simulink model "PIC32MK_MCPWM_MCLV2_PIM_DualShunt_R2015b_InternalOpAmp"  (R2015b)
settings: Solver=FixedStepDiscrete  StartTime=0.0  StopTime=10.0  FixedStep=5e-5  RelTol=1e-3
undefined symbols (not defined in the file): A0, A11, A4, A8, AN0, AN24, AN3, AN9, B1, B6, B9, DiscIntNeverNeededParam, MaxPer, ms, Pin, PWM1max, Resol, us, XData
libraries: MCHP_Blockset x12, simulink x9
(part 1 of 2)
settings Model: Creator=M91449  LastModifiedBy=Lubin Kerhuel
settings DataIOCC: SaveFormat=Array  SignalLoggingSaveFormat=ModelDataLogs
settings OptimizationCC: DefaultParameterBehavior=Inlined  ExpressionDepthLimit=2147483647  OptimizeModelRefInitCode=on  LifeSpan=1
settings DebuggingCC: UnderspecifiedInitializationDetection=Classic  MergeDetectMultiDrivingBlocksExec=none  SolverPrmCheckMsg=warning  FcnCallInpInsideContextMsg=EnableAllAsWarning  StateNameClashWarn=warning
settings HardwareCC: ProdBitPerPointer=32  ProdLargestAtomicInteger=Integer  ProdWordSize=32  ProdLongLongMode=on  ProdHWDeviceType=Generic->Custom
settings ModelReferenceCC: ModelReferenceNumInstancesAllowed=Single
settings RTWCC: SystemTargetFile=MCHP_pic32_stf.tlc  TemplateMakefile=MCHP_pic32.tmf  Description=Microchip Embedded Target PIC32 (real-time)  GenerateReport=on  IncludeHyperlinkInReport=on  LaunchReport=on  GenerateTraceInfo=on  GenerateTraceReport=on  GenerateTraceReportSl=on  GenerateTraceReportSf=on  GenerateTraceReportEml=on  GenerateCodeReplacementReport=on
settings CodeAppCC: ForceParamTrailComments=on  IgnoreCustomStorageClasses=off  MaxIdLength=255  OperatorAnnotations=on  SimulinkDataObjDesc=on  SFDataObjDesc=on  MATLABFcnDesc=on  CustomSymbolStrType=$N$R$M  InsertBlockDesc=on  MATLABSourceComments=on  InternalIdentifier=Classic
settings STFCustomTargetCC: TargetLibSuffix=_lib.a  CodeReplacementLibrary=GNU C99 extensions  ConcurrentExecutionCompliant=off  IncludeMdlTerminateFcn=off  GeneratePreprocessorConditionals=Use local settings  CombineOutputUpdateFcns=on  CombineSignalStateStructs=on  SuppressErrorStatus=on  ERTCustomFileBanners=on  SupportAbsoluteTime=off  SupportNonFinite=off  SupportComplex=off  SupportContinuousTime=off  MATLABClassNameForMDSCustomization=Simulink.SoftwareTarget.ERTCustomization  CPPClassGenCompliant=off  GRTInterface=off  SystemTargetFile=MCHP_pic32_stf.tlc
settings ERTTargetCC: TargetLibSuffix=_lib.a  CodeReplacementLibrary=GNU C99 extensions  ParMdlRefBuildCompliant=off  CompOptLevelCompliant=off  ConcurrentExecutionCompliant=off  IncludeMdlTerminateFcn=off  CombineSignalStateStructs=on  SuppressErrorStatus=on  ERTFirstTimeCompliant=off  SupportAbsoluteTime=off  SupportNonFinite=off  SupportComplex=off  SupportNonInlinedSFcns=on  ModelStepFunctionPrototypeControlCompliant=off  CPPClassGenCompliant=off  UseToolchainInfoCompliant=off  InlinedParameterPlacement=NonHierarchical  ERTSrcFileBannerTemplate=MCHP_dsPIC_code_template.cgt  ERTHdrFileBannerTemplate=MCHP_dsPIC_code_template.cgt  ERTDataSrcFileTemplate=MCHP_dsPIC_code_template.cgt  ERTDataHdrFileTemplate=MCHP_dsPIC_code_template.cgt  ERTCustomFileTemplate=MCHP_main.tlc  ConvertIfToSwitch=on  SuppressUnreachableDefaultCases=on
settings ConfigComp: CovModelRefEnable=Off  CovSFcnEnable=off

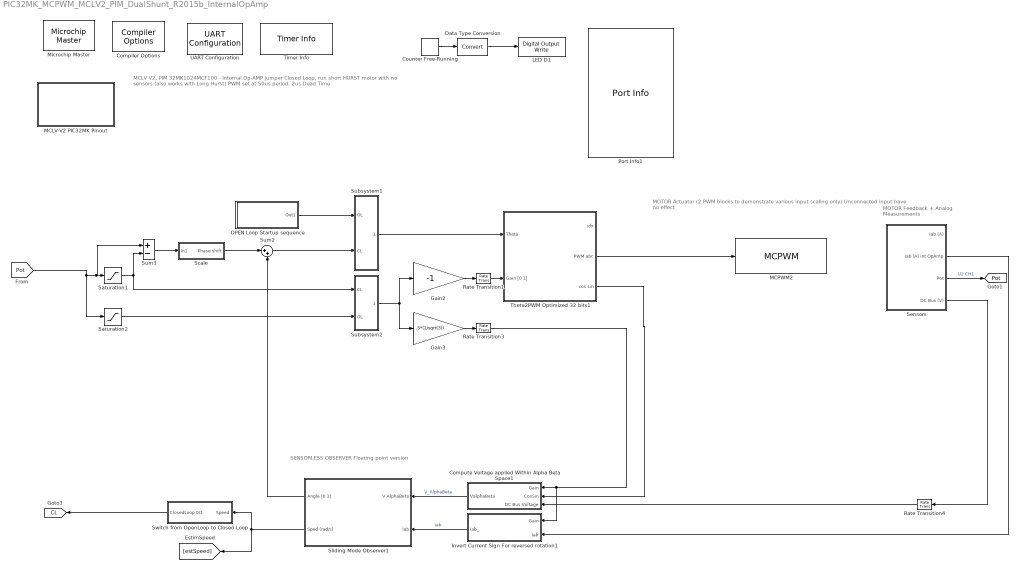
== system PIC32MK_MCPWM_MCLV2_PIM_DualShunt_R2015b_InternalOpAmp ==
  note: MOTOR Feedback
      | + Analog Measurements
  note: MOTOR Actuator (2 PWM blocks to demonstrate various input scaling only)
      | Unconnected input have no effect
  note: MCLV V2, PIM 32MK1024MCF100 - Internal Op-AMP jumper
      |
      | Closed Loop, run short HURST motor with no sensors (also works with Long Hurst)
      | PWM set at 50us period. 2us Dead Time
  note: SENSORLESS OBSERVER
      | Floating point version
  Compiler Options : MCHP_Blockset/System Configuration/Compiler Options  Priority=1  LATEST_CMPLR=on  COMP_LIST=Dynamic Options  COMP_LIST_TXT=xc32 - v2.41  DFP_LIST=Dynamic Options  DFP_LIST_TXT=v 1.4.94  CMSIS_DSP=Dynamic Options  CMSIS_DSP_TXT=Dynamic Options  USE_64BIT_DOUBLE=off  MCHP_MULTITHREAD_COMPILATION=on  UseCustom_LinkerScript=off  MCHP_MASTERLINK=PIC32MK_MCPWM_MCLV2_PIM_DualShunt_R2015b_InternalOpAmp/Microchip Master  OPTIMIZATION_LEVEL=1  OPTIMIZATION_FLTO=on  OPTIMIZATION_REORDER=off  UNROLL_LOOPS=on  PROCEDURAL_ABSTRACTION=off  MPLAB_LINKLIB=default  MPLAB_LINKLIB1=default  MCODE=is less than 32768 (faster)  MCONST=in code memory  MDATA=Use only memory below address 8192 (faster)  MSCALAR=Use only memory below address 8192 (faster)  MLARGEARRAY=off  MAGGREGATE=off  HEAP_SIZE=0  OMF=elf  DEBUG_INFO=on  ProduceHexOutput=on  AssemblyListing=on  NO_EDS_WARN=on  PRINT_STATISTICS=off
  Compute Voltage applied Within Alpha Beta Space1 : Subsystem
  Counter Free-Running : simulink/Sources/Counter Free-Running  NumBits=1  tsamp=.2
  Data Type Conversion : DataTypeConversion
  Gain2 : Gain  Gain=-1  OutMin=-PWM1max*0.5  OutMax=PWM1max*0.5  OutDataTypeStr=double  RndMeth=Zero
  Gain3 : Gain  Gain=.5*(2/sqrt(3))  OutDataTypeStr=double  RndMeth=Zero
  Invert Current Sign For reversed rotation1 : Subsystem
  LED D1 : MCHP_Blockset/Digital IO/Digital Output Write  PORT=Dynamic Options  PORT_TXT="F   [ 0  1  5  6  7  9  10  12  13 ]"  PIN=5  PACK=off  SIMULTANEOUS=off  ORDERING=None  SampleTime=-1  MCHP_PORT={Digital Out}{DOU}1:1:F5;  MCHP_MASTERLINK=PIC32MK_MCPWM_MCLV2_PIM_DualShunt_R2015b_InternalOpAmp/Microchip Master
  MCLV-V2 PIC32MK Pinout : Subsystem
  MCPWM2 : MCHP_Blockset/PWM IO/MCPWM  Priority=-2000  PWMx_ECAM_ITB=Independant - Center aligned - Symetric  PWMx_MTBS=Primary master timer  PWM_ClockResolution=Dynamic Options  PWM_ClockResolution_TXT=auto  MaxPeriod_s=50e-6  InitPeriode_s=50e-6  InitDutyCycleP_s=10e-6  InitDutyCycleS_s=10e-6  InitPhase_s=-1  SampleTime=-1  S_INPUT=[-1]  S_INPUT_Size=[3]  S_OUTPUT=[]  S_OUTPUT_Size=[]  S_ListCustomDatatype=S.S_ListCustomDatatype={};  MCHP_USER_INTERRUPTS=0  evalin_ws=PWM1max=MCHP_Fun.Hex2num('40A7700000000000');PWM2max=MCHP_Fun.Hex2num('40A7700000000000');PWM3max=MCHP_Fun.Hex2num('40A7700000000000');  MCHP_PORT={PWMH1 }{PWMH1}32:4:B14;{PWMH2 }{PWMH2}32:4:B12;{PWMH3 }{PWMH3}32:4:B10;{PWML1}{PWML1}32:4:B15;{PWML2}{PWML2}32:4:B13;{PWML3}{PWML3}32:4:B11;{PWM FLT15}{FLT15}32:0:B4;  MCHP_MASTERLINK=PIC32MK_MCPWM_MCLV2_PIM_DualShunt_R2015b_InternalOpAmp/Microchip Master  MCHP_CRC=3819763  PWMx_PMOD=Complementary  PWM1_HL=PWMxH & PWMxL output enabled  PWM1_swap=off  PWM1H_pol=off  PWM1L_pol=off  PWM2_HL=PWMxH & PWMxL output enabled  PWM2_swap=off  PWM2H_pol=off  PWM2L_pol=off  PWM3_HL=PWMxH & PWMxL output enabled  PWM3_swap=off  PWM3H_pol=off  PWM3L_pol=off  PWM4_HL=not used  PWM4_swap=off  PWM4H_pol=off  PWM4L_pol=off  PWM5_HL=not used  PWM5_swap=off  PWM5H_pol=off  PWM5L_pol=off  PWM6_HL=not used  PWM6_swap=off  PWM6H_pol=off  PWM6L_pol=off  PWM7_HL=not used  PWM7_swap=off  PWM7H_pol=off  PWM7L_pol=off  PWM8_HL=not used  PWM8_swap=off  PWM8H_pol=off  PWM8L_pol=off  PWM9_HL=not used  PWM9_swap=off  PWM9H_pol=off  PWM9L_pol=off  PWM10_HL=not used  PWM10_swap=off  PWM10H_pol=off  PWM10L_pol=off  PWM11_HL=not used  PWM11_swap=off  PWM11H_pol=off  PWM11L_pol=off  PWM12_HL=not used  PWM12_swap=off  PWM12H_pol=off  PWM12L_pol=off  Init_SEVTCMP_SSEVTCMP=-1  Init_TRIGx_STRIGx_1=[1.8e-6 ,-1]  Init_TRIGx_STRIGx_2=[-1 -1]  Init_TRIGx_STRIGx_3=[-1 -1]  Init_TRIGx_STRIGx_4=[-1 -1]  Init_TRIGx_STRIGx_5=[-1 -1]  Init_TRIGx_STRIGx_6=[-1 -1]  Init_TRIGx_STRIGx_7=[-1 -1]  Init_TRIGx_STRIGx_8=[-1 -1]  Init_TRIGx_STRIGx_9=[-1 -1]  Init_TRIGx_STRIGx_10=[-1 -1]  Init_TRIGx_STRIGx_11=[-1 -1]  Init_TRIGx_STRIGx_12=[-1 -1]  TRIG_DualTriggerMode=Primary Trigger to ADC is independant  BlockInput_VectorScalar=Vectors (grouped by function)  BlockInput_Period=Not a block input  BlockInput_DutyCycle=a Floating Point input within range [-1 1]  BlockInput_PhaseShift=Not a block input  BlockInput_SEVTCMP=Not a block input  BlockInput_TRIGx=Not a block input  BlockInput_DeadTime=Not a block input  BlockOutput_FaultDisabled=off  BlockOutput_Fault=off  DTC=Positive dead time (ensure period of time with PWM_H and PWM_L disasserted)  FLTSRC1_DTCMP=Dynamic Options  FLTSRC1_DTCMP_TXT="FLT6 / E13 / Pin[42]  -  Active HIGH"  FLTSRC2_DTCMP=Dynamic Options  FLTSRC2_DTCMP_TXT="FLT6 / E13 / Pin[42]  -  Active LOW"  FLTSRC3_DTCMP=Dynamic Options  FLTSRC3_DTCMP_TXT="FLT8 / E15 / Pin[44]  -  Active LOW"  FLTSRC4_DTCMP=Dynamic Options  FLTSRC4_DTCMP_TXT="FLT3 / C2 / Pin[34]  -  Active HIGH"  FLTSRC5_DTCMP=Dynamic Options  FLTSRC5_DTCMP_TXT="FLT3 / C2 / Pin[34]  -  Active HIGH"  FLTSRC6_DTCMP=Dynamic Options  FLTSRC6_DTCMP_TXT="FLT3 / C2 / Pin[34]  -  Active HIGH"  FLTSRC7_DTCMP=Dynamic Options  FLTSRC7_DTCMP_TXT="FLT3 / C2 / Pin[34]  -  Active HIGH"  FLTSRC8_DTCMP=Dynamic Options  FLTSRC8_DTCMP_TXT="FLT3 / C2 / Pin[34]  -  Active HIGH"  FLTSRC9_DTCMP=Dynamic Options  FLTSRC9_DTCMP_TXT="FLT3 / C2 / Pin[34]  -  Active HIGH"  FLTSRC10_DTCMP=Dynamic Options  FLTSRC10_DTCMP_TXT="FLT3 / C2 / Pin[34]  -  Active HIGH"  FLTSRC11_DTCMP=Dynamic Options  FLTSRC11_DTCMP_TXT="FLT3 / C2 / Pin[34]  -  Active HIGH"  FLTSRC12_DTCMP=Dynamic Options  FLTSRC12_DTCMP_TXT="FLT3 / C2 / Pin[34]  -  Active HIGH"  DeadTime_s=2e-6  DeadTimeAlt_s=2e-6  DeadTimeComp_s=0  FLTMODx=Force PWM output for current cycle. Enable PWM on next cycle  FLTSRCx=Dynamic Options  FLTSRCx_TXT="FLT15 / B4 / Pin[50]  -  Active LOW"  FLTDATx=PWM H/L -> 00  CLMODx=Disabled  CLSRCx=Dynamic Options  CLSRCx_TXT="FLT8 / E15 / Pin[44]  -  Active LOW"  CLDATx=PWM H/L -> 00  FLTLEBENx=off  CLLEBENx=off  LeadEdgeBlkPer_s=5e-7  PHRx=off  PHFx=off  PLRx=off  PLFx=off
  Microchip Master : MCHP_Blockset/System Configuration/Microchip Master  PICREF=32MK1024MCF100  TIMESTEP_REF=PWM1 trigger + ADC  BUSYFLAG=Dynamic Options  BUSYFLAG_TXT=None  PWRTEN=Not used  BOREN=Disable  BODENV=2.7V  BORV=Not used  FPWRT=128ms  DSBOREN=Enable ZPBOR during Deep Sleep Mode  DSLPBOR=Not used  MCLRE=Enabled  SMCLR=MCLR pin generates a normal system Reset  PMDL1WAY=Allow only one reconfiguration  RSTPRI=Device will obtain reset instruction from Primary flash  TEMP=Not used  SOSCSRC=Not used  SOSCSEL=Not used  IOL1WAY=Allow only one reconfiguration  ALTVREF=Not used  DISUVREG=Not used  DSSWEN=Not used  LPCFG=Not used  RTCBAT=Not used  VBTBOR=Not used  WUTSEL=Not used  POWERSAVE=off  FNOSC=Primary Osc (HS;EC)  FPR=ECIO w/ PLL 16x  FOSFPR=HS3 w/PLL 16x  FOS=Primary Oscillator  FRANGE=High Range  OSCILLATOR_SELECT=External Clock  OSCILLATOR_SELECT_spd=External Clock  QUARTZ=24e6  QUARTZ_spd=24e6  POSCGAIN=Gain Level 3 (highest)  POSCBOOST=Boost the kick start of the oscillator  SOSCGAIN=2x gain setting  SOSCBOOST=Boost the kick start of the oscillator  ACTIV_PLL=on  ACTIV_PLL_spd=on  MIPS_DESIRED=120e6  MIPS_DESIRED_spd=120e6  FPLLMUL=Not used  FPLLIDIV=1x Divider  POSCFREQ=Not used  POSCMD=EC (External Clock) Mode  POSCMOD=External clock mode  MIPS=120 * 1e6  ACLKCON=Optimized for PWM resolution & ADC conversion speed  ACLKCON_spd=Optimized for PWM resolution & ADC conversion speed  FPLLODIV=4x Divider  PLLKEN=Clock switch to PLL source will wait until the PLL lock signal is valid.  FCKSM=Clock Switch Enabled; FSCM Enabled  FCKSMEN=Sw Disabled; Mon Disabled  IESO=Enabled  DSWDTPS=1:2^36  FWDTEN=Disable  FWDTWINSZ=Window size is 25%  FWPSA=1:512  FWPSA0=1:128  FWPSB=1:16  WDT=Disable  WDTPOST=1:32768  WDTPRE=1:128  WDTPS=1:32768  WINDIS=Watchdog Timer is in non-Window mode  WWDTEN=Non-Window mode  DSWDTEN=Enable DSWDT during Deep Sleep Mode  DSWDTOSC=Select LPRC as DSWDT Reference clock  FPBDIV=Not used  FSOSCEN=Enable Secondary Oscillator  LPRCSEL=Not used  OSCIOFCN=Not used  OSCIOFNC=Disable  LVRCFG=Not used  PLL_96MHZ=Not used  PLL96MHZ=Not used  PLLDIV=Not used  WDTCLK=Not used  WDTCMX=Not used  WDTWIN=WDT Window is 25% of WDT period  XTCFG=24-32 MHz crystals  XTBST=Boost the kick-start  APL=Aux Flash Code protect is disabled  APLK=Aux Flash Write Protection or Code Protection is Enabled  AWRP=Auxiliary program memory is not write-protected  BSS=No Boot program Flash segment  BWP=Not used  BWRP=Boot Segment may be written  CP=Protection Disabled  EBS=No Boot EEPROM  ESS=No Segment Data EEPROM  GCP=General Segment Code protect is Disabled  GSS=General Segment Code protect is Disabled  GSS0=Not used  GSSK=General Segment Write Protection or Code Protection is Enabled  GWRP=General Segment may be written  PWP=Not used  RBS=No Boot RAM  RSS=No Secure RAM  SSS=No Secure Segment  SWRP=Secure segment may be written  WPCFG=Not used  WPDIS=Not used  WPEND=Not used  WPFP=Not used  ICESEL=Communicate on PGEC2/PGED2  ICS=Communicate on PGEC1 and PGED1  JTAGEN=Disable  COE=Not used  RES=Not used  DEBUG=Debugger is disabled  BACKBUG=Not used  BKBUG=Not used  ALTI2C=I2C mapped to SDA1/SCL1 pins  ALTI2C1=SDA1/SCK1 pins are selected as the I/O pins for I2C1  ALTI2C2=SDA2/SCK2 pins are selected as the I/O pins for I2C2  ALTI2C3=I2C3 mapped to SDA3/SCL3 pins  ALTQIO=QEA1; QEB1; INDX1 are selected as inputs to QEI1  ALTSS1=SS1A is selected as the I/O pin for SPI1  CMPPOL0=Hysteresis is applied to falling edge  CMPPOL1=Hysteresis is applied to falling edge  FCANIO=Not used  FETHIO=Default Ethernet I/O  FMIIEN=MII Enabled  FSRSSEL=Not used  FUSBIDIO=Controlled by the USB Module  FVBUSONIO=Not used  HPOL=PWM module high side output pins have active-high output polarity  HYST0=45 mV Hysteresis  HYST1=45 mV Hysteresis  I2C1SEL=Not used  LPOL=PWM module low side output pins have active-high output polarity  PWMPIN=PWM module pins controlled by PORT register at device Reset  RTCOSC=Not used  UPLLEN=USB PLL Enabled  UPLLIDIV=Not used  ATMOD8=Not used  ALTPMP=Not used  I2C2SEL=Not used  ALTADREF=Not used  ALTCVREF=Not used  PWMLOCK=PWM registers may be written without key sequence  INT_PRIORITY_DMA=0  MCHP_TIMER_RESULT=[ ]  MCHP_PLLRegisters="[34799619         0     16386         3        -1]"  MCHPVAR=MCHP.fcy.MIPS=1.2e+08;MCHP.fcy.SYSCLK=1.2e+08;MCHP.fcy.ADC=1.2e+08;MCHP.fcy.Comparator=1.2e+08;MCHP.fcy.I2C=1.2e+08;MCHP.fcy.SPI=1.2e+08;MCHP.fcy.UART=1.2e+08;MCHP.fcy.Timers=1.2e+08;MCHP.fcy.OC=1.2e+08;MCHP.fcy.IC=1.2e+08;MCHP.fcy.Ports=1.2e+08;MCHP.fcy.QEI=1.2e+08;MCHP.PowerSave=0;MCHP.TimeStepFactor=-20000;MCHP.TimeStep_Timer=-1;MCHP.NTIMERS=9;MCHP.id.name='32MK1024MCF100';MCHP.id.N=reshape([32 1024 100],1,3);MCHP.id.L=reshape({ 'MK','MCF',''},1,3);MCHP.id.Arch=4;MCHP.periph.PPS.reg_RPINRx=reshape(MCHP_Fun.Hex2num('[]'),0,0);MCHP.PPS.PIC32.PeriphInput_ppsGroup=reshape({ 'INT4','T2CK','T6CK','IC4','IC7','IC12','IC15','U3RX','U4CTS','U6RX','SDI1','SDI3','SCK4_in','SDI5','SS6_in','C3RX','REFCLKI','QEA1','HOME2','QEA3','HOME4','QEA5','HOME6','FLT1','23','24','25','26','27','28','29','30','31','INT3','T3CK','T7CK','IC3','IC8','IC11','IC16','U1CTS','U2RX','U5CTS','SDI2','SDI4','SCK4_in','C2RX','QEB1','INDX2','QEB3','INDX4','QEB5','INDX6','FLT2','SCK6_in','21','22','23','24','25','26','27','28','29','30','31','INT2','T4CK','T8CK','IC1','IC5','IC9','IC13','U1RX','U2CTS','U5RX','SS1_in','SS3_in','SS4_in','SS5_in','C1RX','OCFB','INDX1','QEB2','INDX3','QEB4','INDX5','QEB6','21','22','23','24','25','26','27','28','29','30','31','INT1','T5CK','T9CK','IC2','IC6','IC10','IC14','U3CTS','U4RX','U6CTS','SS2_in','SCK3_in','SCK5_in','SDI6','C4RX','OCFA','HOME1','QEA2','HOME3','QEA4','HOME5','QEA6','21','22','23','24','25','26','27','28','29','30','31'},1,132);MCHP.PPS.PIC32.PeriphOutputCode=reshape({ 'NoConnect','U1TX','U2RTS','SDO1','SDO2','OC1','OC7','C2OUT','C4OUT','OC13','10','U5RTS','C1TX','13','SDO3','SCK4_out','SDO5','SS6_out','REFOUT4','PTGTRIGO28','QEI1CNT','QEI5CNT','22','23','24','25','26','27','28','29','30','31','NoConnect','U3RTS','U4TX','SDO1','SDO2','OC2','OC8','C3OUT','OC9','OC12','OC16','U6RTS','C4TX','13','SDO2','SDO4','SDO5','SCK6_out','REFOUT3','PTGTRIGO29','QEI2CNT','QEI6CNT','22','23','24','25','26','27','28','29','30','31','NoConnect','U3TX','U4RTS','SS1_out','4','OC4','OC5','REFOUT1','C5OUT','OC10','OC14','U6TX','C3TX','13','SS3_out','SS4_out','SS5_out','SDO6','REFOUT2','19','QEI3CNT','21','22','23','24','25','26','27','28','29','30','31','NoConnect','U1RTS','U2TX','3','SS2_out','OC3','OC6','C1OUT','10','OC11','OC15','U5TX','C2TX','13','SCK3_out','SDO4','SCK5_out','SDO6','CTPLS','19','QEI4CNT','21','22','23','24','25','26','27','28','29','30','31'},1,128);MCHP.PPS.PIC32.PinInputCode=reshape({ 'A0','B3','B4','B15','B7','C7','C0','C5','A11','D5','G6','F1','E0','A15','CMP1','FHOME1','A1','B5','B1','B11','B8','A8','C8','B12','A12','D6','G7','G0','E1','A14','CMP2','FINDX1','B6','C15','A4','B13','B2','C6','C1','A7','E14','C13','G8','','F0','D4','PTGTRIGO30','FHOME2','B14','C12','B0','B10','B9','C9','C2','C4','E15','C10','G9','G12','G1','D3','PTGTRIGO31','FINDX2'},1,64);MCHP.Rx=reshape([22 24 32 -1 52 87 90 -1 -1 -1 -1 23 25 33 6 53 88 89 -1 -1 -1 -1 -1 26 34 7 -1 -1 -1 -1 -1 -1 -1 -1 27 -1 8 -1 -1 -1 -1 -1 -1 -1 51 50 -1 9 -1 -1 -1 -1 -1 -1 -1 -1 69 -1 82 -1 61 -1 -1 -1 -1 -1 -1 70 77 83 -1 91 10 -1 -1 -1 -1 3 72 78 -1 -1 92 11 -1 -1 -1 -1 49 74 81 68 18 -1 12 -1 -1 -1 -1 -1 76 84 -1 19 28 14 -1 -1 -1 -1 100 93 71 -1 -1 29 17 -1 -1 -1 -1 21 94 35 -1 -1 -1 38 -1 -1 -1 -1 20 98 63 79 41 40 96 -1 -1 -1 -1 -1 99 73 80 42 39 97 -1 -1 -1 -1 66 4 -1 47 43 -1 95 -1 -1 -1 -1 67 5 64 48 44 -1 1 -1 -1 -1 -1],11,16);MCHP.ADC.ANtype=reshape([0 0],1,2);MCHP.ADC.ADCONx=reshape([0 0 0 0 0 0],1,6);MCHP.ADC.ADCHS_0=reshape([0 0],1,2);MCHP.ADC.Flags=reshape([-1 0],1,2);MCHP.ADC.Buffer=reshape([-1 -1],1,2);MCHP.ADC.port=reshape([0 1 16 17 18 19 32 33 34 11 12 43 76 77 78 79 105 104 103 102 73 72 106 111 4 23 8 25 -1 -1 -1 -1 -1 89 90 107 93 92 62 63 64 65 -1 -1 -1 85 14 15 42 44 -1 -1 -1 -1 -1 -1 -1],1,57);MCHP.ADC.port_ALT=reshape([-1 -1 -1 -1],1,4);MCHP.ADC.port_VrefP=90;MCHP.ADC.port_VrefM=89;MCHP.ADC.port_AVdd=-1;MCHP.ADC.port_AVss=-1;MCHP.ADC.ADCDATA=reshape([1 1 1 1 1 1 1 1 1 1 1 1 1 1 1 1 1 1 1 1 1 1 1 1 1 1 1 1 0 0 0 0 0 1 1 1 1 1 1 1 1 1 0 0 0 1 1 1 1 1 1 1 1 1 0 0 0],1,57);MCHP.ADC.HS_SAR.TRGSRC=reshape([0 0 0 0 0 0 0 0 0 0 0 0 0 0 0 0 0 0 0 0 0 0 0 0 0 0],1,26);MCHP.ADC.HS_SAR.nFilters=0;MCHP.ADC.HS_SAR.nDedicatedCore=0;MCHP.ADC.HS_SAR.CALIBRATION=0;MCHP.ADC.HS_SAR.ADCON1L=-1;MCHP.ADC.HS_SAR.ADC_Class3_idxStart=32;MCHP.memory.RAM=0;MCHP.memory.RAM_XBegin=-1;MCHP.memory.RAM_YBegin=-1;MCHP.memory.RAM_dma=reshape([-1 -1],1,2);MCHP.memory.FLASH_ECC=0;MCHP.DMA.Num=8;MCHP.DMA.CNTmax=65535;MCHP.QEI.QEICONx=reshape([49023 49023 49023 49023 49023 49023],1,6);MCHP.QEI.QEItype=6;MCHP.QEI.Port_QEI_INDX=reshape([-1 -1],1,2);MCHP.QEI.Port_QEI_QEA=reshape([-1 -1],1,2);MCHP.QEI.Port_QEI_QEB=reshape([-1 -1],1,2);MCHP.QEI.Port_QEI_UPDN=reshape([-1 -1],1,2);MCHP.INT.Port=reshape([23 32767 32767 32767 32767],1,5);MCHP.PWM_HS.Flags=reshape([0 0 0],1,3);MCHP.PWM.port_FLT=reshape([-1 -1 -1 34 43 76 77 78 79 -1 -1 -1 -1 -1 -1 20 -1 -1 -1 -1 -1 -1 -1 -1 -1 -1 -1 -1 -1 -1 -1 -1 -1],1,33);MCHP.PWM.PWMRef=-1;MCHP.PWM.Flag=0;MCHP.PWM.Port_PWM_l=reshape([31 -1 29 -1 27 -1 7 -1 49 -1 51 -1 -1 -1 -1 -1 -1 -1 -1 -1 81 -1 54 -1],2,12);MCHP.PWM.Port_PWM_h=reshape([30 -1 28 -1 26 -1 10 -1 50 -1 52 -1 31 -1 29 -1 27 -1 7 -1 80 -1 53 -1],2,12);MCHP.PWM_HS_FEP.nEVTOUT=-1;MCHP.IC.Port=reshape([32767 32767 32767 32767 32767 32767 32767 32767 32767 32767 32767 32767 32767 32767 32767 32767],1,16);MCHP.IC.type=2;MCHP.OC.Port=reshape([32767 32767 32767 32767 32767 32767 32767 32767 32767 32767 32767 32767 32767 32767 32767 32767],1,16);MCHP.OC.type=2;MCHP.CN.Port=reshape([-1 -1 -1 -1 -1 -1 -1 -1 -1 -1 -1 -1 -1 -1 -1 -1 -1 -1 -1 -1 -1 -1 -1 -1 -1 -1 -1 -1 -1 -1 -1 -1 -1 -1 -1 -1 -1 -1 -1 -1 -1 -1 -1 -1 -1 -1 -1 -1 -1 -1 -1 -1 -1 -1 -1 -1 -1 -1 -1 -1 -1 -1 -1 -1 -1 -1 -1 -1 -1 -1 -1 -1 -1 -1 -1 -1 -1 -1 -1 -1 -1 -1 -1 -1 -1],1,85);MCHP.CN.PullUp=reshape([56723 65535 65479 61822 62211 14051 65475 0 0 0 0],1,11);MCHP.CN.type=2;MCHP.CN.Flag_PullDown=1;MCHP.SPI.Refs=reshape([1 2 3 4 5 6],1,6);MCHP.SPI.SPIxCON1=MCHP_Fun.Hex2num('41EFF07FFFE00000');MCHP.SPI.SPIxCON2=40843;MCHP.SPI.Port_SDI=reshape([-1 -1 -1 -1 -1 -1],1,6);MCHP.SPI.Port_SDO=reshape([-1 -1 -1 -1 -1 -1],1,6);MCHP.SPI.Port_SCK=reshape([23 22 -1 -1 -1 -1],1,6);MCHP.SPI.Port_SS=reshape([-1 -1 -1 -1 -1 -1],1,6);MCHP.I2C.Refs=reshape([1 2 3 4 0],1,5);MCHP.I2C.I2CxCON=8388607;MCHP.I2C.NewRegName=1;MCHP.I2C.Port_SDA=reshape([-1 -1 -1 -1 -1],1,5);MCHP.I2C.Port_SCL=reshape([-1 -1 -1 -1 -1],1,5);MCHP.I2C.Port_ASDA=reshape([-1 -1 -1 -1 -1],1,5);MCHP.I2C.Port_ASCL=reshape([-1 -1 -1 -1 -1],1,5);MCHP.I2C.Fuse_Port_SCL_SDA=reshape([-1 -1 -1 -1 -1 -1 -1 -1 -1 -1],2,5);MCHP.I2C.Fuse_Port_ASCL_ASDA=reshape([-1 -1 -1 -1 -1 -1 -1 -1 -1 -1],2,5);MCHP.SCCP.nSCCP=0;MCHP.SCCP.MCCP=reshape([0 0 0 0 0 0 0 0 0],1,9);MCHP.PGA.Port_PGA1P=reshape([-1 -1 -1 -1],1,4);MCHP.PGA.Port_PGA1N=reshape([-1 -1 -1 -1],1,4);MCHP.PGA.Port_PGA2P=reshape([-1 -1 -1 -1],1,4);MCHP.PGA.Port_PGA2N=reshape([-1 -1 -1 -1],1,4);MCHP.PGA.Num=0;MCHP.HS_AnalogComparator.Port_CMP1=reshape([-1 -1 -1 -1],1,4);MCHP.HS_AnalogComparator.Port_CMP2=reshape([-1 -1 -1 -1],1,4);MCHP.HS_AnalogComparator.Port_CMP3=reshape([-1 -1 -1 -1],1,4);MCHP.HS_AnalogComparator.Port_CMP4=reshape([-1 -1 -1 -1],1,4);MCHP.HS_AnalogComparator.PORT_EXTREFx=reshape([-1 -1],1,2);MCHP.HS_AnalogComparator.Port_DACOUTx=reshape([-1 -1],1,2);MCHP.HS_AnalogComparator.Num=0;MCHP.Comp.Port_CVrefin=-1;MCHP.Comp.Port_CVref=-1;MCHP.Comp.Port_CVref1O=-1;MCHP.Comp.Port_CVref2O=-1;MCHP.Comp.Port_CxOUT=reshape([32767 32767 32767 32767 32767],1,5);MCHP.Comp.Port_OAxOUT=reshape([17 0 32 -1 23],1,5);MCHP.Comp.Port_CxINP=reshape([18 1 34 32 4],1,5);MCHP.Comp.Port_CxINM=reshape([19 43 18 17 16 76 18 0 33 77 34 32 33 17 0 32 25 76 4 23],4,5);MCHP.Comp.Port_OAxINP=reshape([18 1 34 -1 4],1,5);MCHP.Comp.Port_OAxINM=reshape([19 16 33 -1 25],1,5);MCHP.Comp.nComp=reshape([5 0 0],1,3);MCHP.Comp.OpAmp=23;MCHP.Comp.CVRCON=reshape([0 0],1,2);MCHP.Comp.CMCON=0;MCHP.CDAC.Port_DACx=reshape([4 42 8],1,3);MCHP.CDAC.nCDAC=3;MCHP.UART.port_Rx=reshape([32767 32767 32767 32767 32767 32767],1,6);MCHP.UART.port_Tx=reshape([32767 32767 32767 32767 32767 32767],1,6);MCHP.UART.port_ARx=reshape([-1 -1],1,2);MCHP.UART.port_ATx=reshape([-1 -1],1,2);MCHP.UART.port_RTS=reshape([32767 32767 32767 32767 32767 32767],1,6);MCHP.UART.port_CTS=reshape([32767 32767 32767 32767 32767 32767],1,6);MCHP.UART.reg_UxMODE=reshape([13106175 13106175 13106175 13106175 13106175 13106175],1,6);MCHP.UART.reg_UxSTA=reshape(MCHP_Fun.Hex2num('[41EFFFFFFFE00000 41EFFFFFFFE00000 41EFFFFFFFE00000 41EFFFFFFFE00000 41EFFFFFFFE00000 41EFFFFFFFE00000]'),1,6);MCHP.modsrc.DOS_02551_cpu_16bit_v7=0;MCHP.modsrc.DOS_01520_wdt_dmt_upb_v1_16bit=0;MCHP.modsrc.DOS_02359a_sent_j2716_upb_v1=0;MCHP.modsrc.DOS_02672_math_progcrc_upb_v1_16bit=0;MCHP.modsrc.DOS_01577_cla_clc_upb_v1=0;MCHP.modsrc.DOS_02915_ecc_v2=0;MCHP.modsrc.DOS_02673_tmr_classa_upb_v1_16bit=0;MCHP.modsrc.DOS_01494_qei_32b_upb_v1_16bit=0;MCHP.modsrc.DOS_02552_msi_upb_v1_Master=0;MCHP.modsrc.DOS_01441_i2c_upb_v1_16bit_TLAH=0;MCHP.modsrc.DOS_03076_uart_protocol_upb_v1_16bit=0;MCHP.modsrc.DOS_01482=0;MCHP.modsrc.DOS_01483_pwm_16bit=0;MCHP.modsrc.DOS_02497_WACV=0;MCHP.modsrc.DOS_02316_nvm_ctrl_v1_16bit=0;MCHP.modsrc.DOS_02653_afe_current_bias_ctrl_upb_v1_16bit=0;MCHP.modsrc.DOS_01459_ptg_pc_upb_v1_16bit=0;MCHP.modsrc.DOS_01512_ccp_mccp_upb_v1_16bit=0;MCHP.modsrc.DOS_02519_dma_sfr_16bit_v2=0;MCHP.modsrc.DOS_02508c11=0;MCHP.modsrc.DOS_02475_dac_pdm_nbit_upb_v1_16bit=0;MCHP.modsrc.DOS_02467_gpio_upb_v1_16bit=0;MCHP.modsrc.DOS_00805_rst_integration_v4=0;MCHP.modsrc.DOS_02659_clk_sib_v12=0;MCHP.modsrc.DOS_02674_wdt_upb_v1_16bit=0;MCHP.modsrc.DOS_01407=0;MCHP.modsrc.DOS_02552_msi_upb_v1_Slave=0;MCHP.modsrc.DOS_02593_amp_pga_ctrl_pb_v2_16bit=0;MCHP.modsrc.DOS_03247_CAN_FD_UPB_V2_16_bit=0;MCHP.modsrc.DOS_01461_afe_ctmu_con_upb_v1_16bit=0;MCHP.modsrc.DOS_02497_WACA=0;MCHP.modsrc.DOS_02478_uart_irda_upb_v1_16bit=0;MCHP.modsrc.DOS_00929=0;MCHP.modsrc.DOS_01198=0;MCHP.modsrc.DOS_03029_WACH=0;MCHP.modsrc.DOS_02949_WACG=0;MCHP.modsrc.DOS_03349_amp_pad_opamp_ctrl_upb_v1=0;MCHP.modsrc.DOS_02237_osc_dco_ctrl_upb_v1_16bit=0;MCHP.modsrc.DOS_02472_ppi_pmp16_upb_v1_16bit=0;MCHP.modsrc.DOS_03994_WAC07=0;MCHP.modsrc.DOS_03662_WACU=0;MCHP.modsrc.DOS_00794=0;MCHP.modsrc.DOS_00931=0;MCHP.modsrc.DOS_00932=0;MCHP.modsrc.DOS_00942=0;MCHP.modsrc.DOS_00938=0;MCHP.modsrc.DOS_00996=0;MCHP.modsrc.DOS_00997=0;MCHP.modsrc.DOS_00998=0;MCHP.modsrc.DOS_00209=0;MCHP.modsrc.DOS_01555_adc=0;MCHP.modsrc.DOS_01293=0;MCHP.modsrc.DOS_00828=0;MCHP.modsrc.DOS_01116=0;MCHP.modsrc.DOS_01017_RPORx=0;MCHP.modsrc.DOS_01017_RPINRx=0;MCHP.modsrc.DOS_01555_nvm_tsmc18_v2_16bit=0;MCHP.modsrc.DOS_00804=0;MCHP.modsrc.DOS_00826=0;MCHP.modsrc.DOS_01555_TLAK_PMDx=0;MCHP.modsrc.DOS_01555_TLAK_INT_=0;MCHP.modsrc.DOS_00933=0;MCHP.modsrc.DOS_01555=0;MCHP.modsrc.DOS_01555_ptg=0;MCHP.modsrc.DOS_00958=0;MCHP.modsrc.DOS_01117_PORTx=0;MCHP.modsrc.DOS_00999=0;MCHP.modsrc.DOS_01041=0;MCHP.modsrc.DOS_00892=0;MCHP.modsrc.DOS_01287_TLAC_PMDx=0;MCHP.modsrc.DOS_01287_TLAC_INT_=0;MCHP.modsrc.DOS_01424=0;MCHP.modsrc.DOS_01332=0;MCHP.modsrc.DOS_01468_PMBA_current_source=0;MCHP.modsrc.DOS_02291_PGA=0;MCHP.modsrc.DOS_01467_Comparator=0;MCHP.modsrc.DOS_01498_TLAY=0;MCHP.modsrc.DOS_00993_PLL_120MHz=0;MCHP.modsrc.DOS_01332_ptg_pc_v1=0;MCHP.modsrc.DOS_00958_pwm_TLAY=0;MCHP.modsrc.TLAY_IOPorts=0;MCHP.modsrc.DOS_00929q=0;MCHP.modsrc.DOS_02415_spi_v5=0;MCHP.modsrc.DOS_RPINRx_16bit_2=0;MCHP.modsrc.DOS_01497_TLAH_PMDx=0;MCHP.modsrc.DOS_02550_TLAL_INT=0;MCHP.modsrc.DOS_00958_pwm_TLAH=0;MCHP.modsrc.DOS_01287_TLAH_INT_=0;MCHP.modsrc.DOS_01113=0;MCHP.modsrc.DOS_01017_PMDx=0;MCHP.modsrc.DOS_00927=0;MCHP.modsrc.DOS_01080=0;MCHP.modsrc.DOS_00794_cpu_16bit_v3=0;MCHP.modsrc.DOS_02192_TLCD_PMDx=0;MCHP.modsrc.DOS_02192_TLCD_INT_=0;MCHP.modsrc.DOS_02192_cmp=0;MCHP.modsrc.DOS_00958_pwm_TLCD=0;MCHP.modsrc.DOS_02192_PORTx_TLCD=0;MCHP.modsrc.DOS_00936=0;MCHP.modsrc.DOS_00995=0;MCHP.modsrc.DOS_00546=0;MCHP.modsrc.DOS_00474=0;MCHP.modsrc.DOS_02481_WACJ_MC_Config=1;MCHP.modsrc.DOS_02569_pfm_cache_ocp_v1=1;MCHP.modsrc.DOS_02819_pfm_ctrl_32bit_upb_v2=1;MCHP.modsrc.DOS_02674_wdt_upb_v1_32bit=1;MCHP.modsrc.DOS_01520_wdt_dmt_upb_v1=1;MCHP.modsrc.DOS_02869_icd_jtag_bvci_upb_v2=1;MCHP.modsrc.DOS_02823_WACJ_clk_cru_upb_v2=1;MCHP.modsrc.DOS_01423_RPINRx=1;MCHP.modsrc.DOS_02481_RPORx=1;MCHP.modsrc.DOS_02511_pwr_sib_upb_v1_32bit=1;MCHP.modsrc.DOS_02481_WACJ_MC_int_evic_v3=1;MCHP.modsrc.DOS_01500_dma_bvci_v2=1;MCHP.modsrc.DOS_02141_tmr_classa_pb_v2=1;MCHP.modsrc.DOS_02815_tmr_classb_upb_v1=1;MCHP.modsrc.DOS_00740_icap_pb_v1=1;MCHP.modsrc.DOS_00749_ocmp_pb_v1=1;MCHP.modsrc.DOS_01441_i2c_upb_v1_32bit=1;MCHP.modsrc.DOS_01329_spi_pb_v2=1;MCHP.modsrc.DOS_02478_uart_irda_upb_v1_32bit=1;MCHP.modsrc.DOS_02514_dfm_strl_sst_upb_v1=1;MCHP.modsrc.DOS_01477_pwm_mc_upb_v1=1;MCHP.modsrc.DOS_01459_ptg_pc_upb_v1_SIC=1;MCHP.modsrc.DOS_01494_qei_32b_upb_v1=1;MCHP.modsrc.DOS_01427_cmp_control_upb_v1_32bit=1;MCHP.modsrc.DOS_01445_dac_nbit__control_upb_v1_32bit=1;MCHP.modsrc.DOS_01461_afe_ctmu_con_upb_v1=1;MCHP.modsrc.DOS_02472_ppi_pmp16_upb_v1=1;MCHP.modsrc.DOS_02467_gpio_ports_upb_v1=1;MCHP.modsrc.DOS_01152_can_bvci_v1=1;MCHP.modsrc.DOS_02508_adc_sar_ctrl_upb_v1_PIC32MK=1;MCHP.modsrc.DOS_02813a_usb_otgcore_pb_v3=1;MCHP.modsrc.DOS_01261_tmr_rtcc_pb_v2=1;MCHP.modsrc.DOS_01475_lpwr_deep_sleep_ctrl_v2=1;MCHP.modsrc.DOS_EIP_00136_ssx_v1=1;MCHP.modsrc.DOS_02481_WACK_MC_Config=0;MCHP.modsrc.DOS_03088_pfm_cache_ocp_v2_WACK=0;MCHP.modsrc.DOS_02823_WACN_clk_cru_upb_v2=0;MCHP.modsrc.DOS_02907_WACK_MC_int_evic_v3=0;MCHP.modsrc.DOS_03554_cmp_control_upb_v2_32bit=0;MCHP.modsrc.DOS_03247_can_fd_upb_v2_pic32mk=0;MCHP.modsrc.DOS_02787_WACD_Config=0;MCHP.modsrc.DOS_00800_dac_4bit_ctrl_pb_v1=0;MCHP.modsrc.DOS_01539_icd_jtag_pb_v2=0;MCHP.modsrc.DOS_02823_clk_cru_upb_v2=0;MCHP.modsrc.DOS_01423_RPORx=0;MCHP.modsrc.DOS_02907_WACD_int_evic_v3=0;MCHP.modsrc.DOS_00734_uart_irda_pb_v1=0;MCHP.modsrc.DOS_00687_tmr_classa_pb_v1=0;MCHP.modsrc.DOS_00745_tmr_classb_pb_v1=0;MCHP.modsrc.DOS_02508_adc_sar_ctrl_upb_v1=0;MCHP.modsrc.DOS_00866_cmp_control_pb_v2=0;MCHP.modsrc.DOS_01114_eth_bvci_v1=0;MCHP.modsrc.DOS_02831_usb_clk_rst_v2=0;MCHP.modsrc.DOS_01643_pfm_cache_ahb_v2=0;MCHP.modsrc.DOS_EIP_00206r5_sqi_v2=0;MCHP.modsrc.DOS_EIP_00124_usb_hs_otgcore_v1=0;MCHP.modsrc.DOS_EIP_00218_math_rng_ahbs_v2=0;MCHP.modsrc.DOS_EIP_00109_ebi_v1=0;MCHP.modsrc.DOS_EIP_00158_crypto_v1=0;MCHP.PortBase=16;MCHP.PortPrefixe='P';MCHP.clock.PBxDIV=reshape([0 0 0 0 0 3 0 -1],1,8);  MCHP_CRC=15127327  BTMODE=Not used  RES1=Not used  PLLSS=Not used  RES2=Not used  ALTCMPI=Not used  BOREN1=Not used  ALTRB6=Not used  RETCFG=Not used  DFMCY=Not used  BSS2=No Boot Segment  BSEN=No Boot Segment  CWRP=Configuration Segment may be written  CSS=No Protection (other than CWRP)  AIVTDIS=Disable Alternate Vector Table  BSLIM=Not used  WDTEN=Disable  BTSWP=BOOTSWP instruction is disabled  DBCC=No Cross Connection between DAC outputs  CTXT1=Not Assigned  CTXT2=Not Assigned  SEQNUM=Not used  nSEQNUM=Not used  BOREN0=Enabled  DMTIVT=Not used  DMTCNT=2^31 (2147483648)  DMTEN=Dead Man Timer is Enabled and cannot be disabled by software  ON=Not used  USERID=Not used  RESERVED1=Not used  PGL1WAY=Allow only one reconfiguration  FPLLRNG=13-26 MHz Input  FPLLICLK=POSC is input to the System PLL  FPLLMULT=PLL Multiply by 20  UPLLFSEL=USB PLL input is 24 MHz  DMTINTV=Window/Interval value is 127/128 counter value  WDTSPGM=WDT stops during Flash programming  FDMTEN=Deadman Timer is disabled  TRCEN=Trace features in the CPU are enabled  BOOTISA=Boot code and Exception code is MIPS32  FECCCON=ECC and Dynamic ECC are disabled (ECCCON bits are writable)  EXTDDRSIZE=Not used  FSLEEP=Flash is powered down when the device is in Sleep mode  DBGPER=Allow CPU access to all permission regions  EJTAGBEN=Normal EJTAG functionality  TSEQ=Not used  CSEQ=Not used  RWDTPS=1:1048576  RCLKSEL=Always use LPRC  SWDTPS=1:1048576  DMTIVTL=Not used  DMTIVTH=Not used  DMTCNTL=Not used  DMTCNTH=Not used  DMTDIS=Dead Man Timer is Disabled and can be enabled by software  SMBEN=SMBus input threshold is enabled  SPI2PIN=SPI2 uses I/O remap (PPS) pins  CTXT3=Not Assigned  CTXT4=Not Assigned  MBXM0=Mailbox register configured for Master data read (Slave to Master data transfer)  MBXM1=Mailbox register configured for Master data read (Slave to Master data transfer)  MBXM2=Mailbox register configured for Master data read (Slave to Master data transfer)  MBXM3=Mailbox register configured for Master data read (Slave to Master data transfer)  MBXM4=Mailbox register configured for Master data read (Slave to Master data transfer)  MBXM5=Mailbox register configured for Master data read (Slave to Master data transfer)  MBXM6=Mailbox register configured for Master data read (Slave to Master data transfer)  MBXM7=Mailbox register configured for Master data read (Slave to Master data transfer)  MBXM8=Mailbox register configured for Master data read (Slave to Master data transfer)  MBXM9=Mailbox register configured for Master data read (Slave to Master data transfer)  MBXM10=Mailbox register configured for Master data read (Slave to Master data transfer)  MBXM11=Mailbox register configured for Master data read (Slave to Master data transfer)  MBXM12=Mailbox register configured for Master data read (Slave to Master data transfer)  MBXM13=Mailbox register configured for Master data read (Slave to Master data transfer)  MBXM14=Mailbox register configured for Master data read (Slave to Master data transfer)  MBXM15=Mailbox register configured for Master data read (Slave to Master data transfer)  MBXHSA=MSIxMBXD15 assigned to mailbox handshake protocol block A  MBXHSB=MSIxMBXD15 assigned to mailbox handshake protocol block B  MBXHSC=MSIxMBXD15 assigned to mailbox handshake protocol block C  MBXHSD=MSIxMBXD15 assigned to mailbox handshake protocol block D  MBXHSE=MSIxMBXD15 assigned to mailbox handshake protocol block E  MBXHSF=MSIxMBXD15 assigned to mailbox handshake protocol block F  MBXHSG=MSIxMBXD15 assigned to mailbox handshake protocol block G  MBXHSH=MSIxMBXD15 assigned to mailbox handshake protocol block H  HSAEN=Mailbox data flow control handshake protocol block disabled.  HSBEN=Mailbox data flow control handshake protocol block disabled.  HSCEN=Mailbox data flow control handshake protocol block disabled.  HSDEN=Mailbox data flow control handshake protocol block disabled.  HSEEN=Mailbox data flow control handshake protocol block disabled.  HSFEN=Mailbox data flow control handshake protocol block disabled.  HSGEN=Mailbox data flow control handshake protocol block disabled.  HSHEN=Mailbox data flow control handshake protocol block disabled.  CPRA0=Master core owns pin.  CPRA1=Master core owns pin.  CPRA2=Master core owns pin.  CPRA3=Master core owns pin.  CPRA4=Master core owns pin.  CPRB0=Master core owns pin.  CPRB1=Master core owns pin.  CPRB2=Master core owns pin.  CPRB3=Master core owns pin.  CPRB4=Master core owns pin.  CPRB5=Master core owns pin.  CPRB6=Master core owns pin.  CPRB7=Master core owns pin.  CPRB8=Master core owns pin.  CPRB9=Master core owns pin.  CPRB10=Master core owns pin.  CPRB11=Master core owns pin.  CPRB12=Master core owns pin.  CPRB13=Master core owns pin.  CPRB14=Master core owns pin.  CPRB15=Master core owns pin.  CPRC0=Master core owns pin.  CPRC1=Master core owns pin.  CPRC2=Master core owns pin.  CPRC3=Master core owns pin.  CPRC4=Master core owns pin.  CPRC5=Master core owns pin.  CPRC6=Master core owns pin.  CPRC7=Master core owns pin.  CPRC8=Master core owns pin.  CPRC9=Master core owns pin.  CPRC10=Master core owns pin.  CPRC11=Master core owns pin.  CPRC12=Master core owns pin.  CPRC13=Master core owns pin.  CPRC14=Master core owns pin.  CPRC15=Master core owns pin.  CPRD0=Master core owns pin.  CPRD1=Master core owns pin.  CPRD2=Master core owns pin.  CPRD3=Master core owns pin.  CPRD4=Master core owns pin.  CPRD5=Master core owns pin.  CPRD6=Master core owns pin.  CPRD7=Master core owns pin.  CPRD8=Master core owns pin.  CPRD9=Master core owns pin.  CPRD10=Master core owns pin.  CPRD11=Master core owns pin.  CPRD12=Master core owns pin.  CPRD13=Master core owns pin.  CPRD14=Master core owns pin.  CPRD15=Master core owns pin.  CPRE0=Master core owns pin.  CPRE1=Master core owns pin.  CPRE2=Master core owns pin.  CPRE3=Master core owns pin.  CPRE4=Master core owns pin.  CPRE5=Master core owns pin.  CPRE6=Master core owns pin.  CPRE7=Master core owns pin.  CPRE8=Master core owns pin.  CPRE9=Master core owns pin.  CPRE10=Master core owns pin.  CPRE11=Master core owns pin.  CPRE12=Master core owns pin.  CPRE13=Master core owns pin.  CPRE14=Master core owns pin.  CPRE15=Master core owns pin.  S1FNOSC=Internal Fast RC (FRC) Oscillator with postscaler  S1IESO=Start up with FRC; then switch  S1OSCIOFNC=OSC2 is clock output  S1FCKSM=Both Clock switching and Fail-safe Clock Monitor are disabled  S1PLLKEN=S1PLLKEN_ON  S1RWDTPS=1:1048576  S1RCLKSEL=Always use LPRC  S1WINDIS=Watchdog Timer operates in Non-Window mode  S1WDTWIN=WDT Window is 25% of WDT period  S1SWDTPS=1:1048576  S1FWDTEN=Disable  S1ICS=Communicate on PGC1 and PGD1  S1DEBUG=Not used  S1ISOLAT=The slave can operate (in debug mode) even if the SLVEN bit in the MSI is zero.  S1NOBTSWP=BOOTSWP instruction is disabled  S1ALTI2C1=I2C1 mapped to SDA1/SCL1 pins  S1SPI1PIN=Slave SPI1 uses I/O remap (PPS) pins  S1SSRE=Slave generated resets will reset the Slave Enable Bit in the MSI module  S1MSRE=The master software oriented RESET events (RESET Op-Code; Watchdog timeout; TRAP reset; illegalInstruction) will also cause the slave subsystem to reset.  S1CTXT1=Not Assigned  S1CTXT2=Not Assigned  S1CTXT3=Not Assigned  S1CTXT4=Not Assigned  BORLVL=Not used  BSSO=Not used  MCA=Not used  MAXTEMP=Not used  CFGAN14=Not used  CFGAN15=Not used  S1IOL1WAY=Not used  S1BSSO=Not used  S1BACKBUG=Not used  BISTDIS=mBIST on reset feature disabled  NOBTSWP=BOOTSWP instruction is disabled  S1BISTDIS=Slave BIST on reset feature disabled  S1DMTIVTL=Not used  S1DMTIVTH=Not used  S1DMTCNTL=Not used  S1DMTCNTH=Not used  S1DMTDIS=Slave Dead Man Timer is Disabled and can be enabled by software  BSEQ=Not used  IBSEQ=Not used  SMB3EN=SMBus 3.0 input levels  FUSBIDIO2=USBID pin is controlled by the USB2 module  FVBUSIO2=VBUSON pin is controlled by the USB2 module  FUSBIDIO1=USBID pin is controlled by the USB1 module  FVBUSIO1=VBUSON pin is controlled by the USB1 module  VBATBOREN=Enable ZPBOR during VBAT Mode  FDSEN=Enable DSEN bit in DSCON  BORSEL=BOR trip voltage 2.1v (Non-OPAMP deviced operation)  POSCFGAIN=Gain is G3  POSCAGCDLY=Settling time = 25ms x AGCRNG  POSCAGCRNG=Range 1x  POSCAGC=Automatic Gain Control for Oscillator  FDBGWP=Not used
  OPEN Loop Startup sequence : Subsystem
  Port Info1 : MCHP_Blockset/System Info/Port Info  MCHP_MASTERLINK=PIC32MK_MCPWM_MCLV2_PIM_DualShunt_R2015b_InternalOpAmp/Microchip Master
  Rate Transition1 : RateTransition
  Rate Transition3 : RateTransition
  Rate Transition4 : RateTransition  Deterministic=off
  Saturation1 : Saturate  UpperLimit=sqrt(3)/2 * (49/50)  LowerLimit=-sqrt(3)/2 * (49/50)
  Saturation2 : Saturate  UpperLimit=0.84*.3  LowerLimit=-0.84*.3
  Scale : Subsystem
  Sensors : Subsystem
  Sliding Mode Observer1 : Subsystem
  Subsystem1 : Subsystem
  Subsystem2 : Subsystem
  Sum2 : Sum  Inputs=|++
  Sum3 : Sum  Inputs=+-
  Switch from OpenLoop to Closed Loop : Subsystem
  Theta2PWM Optimized 32 bits1 : Subsystem  VariantControl=Optimized
  Timer Info : MCHP_Blockset/System Info/Timer Info  MCHP_MASTERLINK=PIC32MK_MCPWM_MCLV2_PIM_DualShunt_R2015b_InternalOpAmp/Microchip Master
  UART Configuration : MCHP_Blockset/BUS UART/UART Configuration  UART_REF=2  BAUD_Choice=Dynamic Options  BAUD_Choice_TXT="6000000         [+0.00%]"  BAUD_Choice_IR=Dynamic Options  BAUD_Choice_IR_TXT=[]  BAUD_Custom=115200  INT_PRIORITY=0  ALT_IO=on  PIN_RX=Dynamic Options  PIN_RX_TXT=A8 / Pin[49]  PIN_TX=Dynamic Options  PIN_TX_TXT=B9 / Pin[76]  MCHP_PORT="{UART2  Rx}{U2RX}3:0:P8;{UART2  Tx}{U2TX}3:1:P25;"  MCHP_MASTERLINK=PIC32MK_MCPWM_MCLV2_PIM_DualShunt_R2015b_InternalOpAmp/Microchip Master  MCHP_COM_ExtPil=off  TX_IMPLEMENTATION=Circular Buffer  TX_IMPLEMENTATION_default=Circular Buffer  TX_INT_PRIORITY=5  TX_INT_WHEN=is empty & last char is sent  TX_INT_WHEN_default=is empty & last char is sent  TX_CIRCULAR_SIZE=256  TX_DMA_CHANNEL="0   (Lowest Priority)"  TX_DMA_SIZE=[]  TX_TASK_PROTECTION=Delay tasks (default)  TX_INTERRUPT_PROTECTION=Do not send on conflict (default)  TX_INTERRUPT_PROTECTION_default=Do not send on conflict (default)  RX_IMPLEMENTATION=Circular Buffer  RX_IMPLEMENTATION_default=Circular Buffer  RX_INT_PRIORITY=1  RX_INT_WHEN=receive 1 character  RX_CIRCULAR_SIZE=256  RX_DMA_CHANNEL=0  RX_DMA_SIZE=0  DuplexMode=Full duplex (default)  PIN_RX_Inv=off  PIN_TX_Inv=off  PIN_RXTX_Inv=off  ParityBit=No parity (default)  StopBit=1 stop bit (default)  IRDA=off  FlowControl=None  PIN_CTS=Dynamic Options  PIN_CTS_TXT=B6 / Pin[70]  PIN_RTS=Dynamic Options  PIN_RTS_TXT=A0 / Pin[22]  InitSequence_chkbox=off  BAUD_Choice_InitSeq=Dynamic Options  BAUD_Choice_InitSeq_TXT="110         [+4.04%]"  BAUD_Choice_IR_InitSeq=Dynamic Options  BAUD_Choice_IR_InitSeq_TXT=0  BAUD_Custom_InitSeq=0  InitSequence='Hello World'
  tag scope: CL=global, Pot=global
  wires:
  Theta2PWM Optimized 32 bits1/2(PWM abc) -> MCPWM2/1
  Sliding Mode Observer1/2(Sped (rad/s)) -> Switch from OpenLoop to Closed Loop/1(Speed), [estSpeed]
  Sliding Mode Observer1/1(Angle [0 1]) -> Sum2/2
  Sensors/3(Pot) -> [Pot]  "U2 CH1"
  Subsystem1/1(OL/CL) -> Theta2PWM Optimized 32 bits1/1(Theta)
  Subsystem2/1(OL/CL) -> Gain2/1, Gain3/1
  Gain2/1 -> Rate Transition1/1
  Gain3/1 -> Rate Transition3/1
  Saturation1/1 -> Sum3/2, Subsystem2/1(CL)
  Saturation2/1 -> Subsystem2/2(OL)
  Rate Transition1/1 -> Theta2PWM Optimized 32 bits1/2(Gain [0 1])
  Switch from OpenLoop to Closed Loop/1(ClosedLoop 0/1) -> [CL]
  [Pot] -> Saturation2/1, Sum3/1, Saturation1/1
  Sum2/1 -> Subsystem1/2(CL)
  OPEN Loop Startup sequence/1(Out1) -> Subsystem1/1(OL)
  Sum3/1 -> Scale/1(In1)
  Scale/1(Phase shift) -> Sum2/1
  Counter Free-Running/1 -> Data Type Conversion/1
  Data Type Conversion/1 -> LED D1/1
  Invert Current Sign For reversed rotation1/1("Iab_ ") -> Sliding Mode Observer1/2(Iab)  "Iab"
  Compute Voltage applied Within Alpha Beta Space1/1(ValphaBeta) -> Sliding Mode Observer1/1(V AlphaBeta)  "V_AlphaBeta"
  Rate Transition3/1 -> Invert Current Sign For reversed rotation1/1(Gain), Compute Voltage applied Within Alpha Beta Space1/1(Gain)
  Theta2PWM Optimized 32 bits1/3(cos sin) -> Compute Voltage applied Within Alpha Beta Space1/2(CosSin)
  Rate Transition4/1 -> Compute Voltage applied Within Alpha Beta Space1/3(DC Bus Voltage)
  Sensors/2(Iab (A) int OpAmp) -> Invert Current Sign For reversed rotation1/2("Iab ")
  Sensors/4(DC Bus (V)) -> Rate Transition4/1

== system PIC32MK_MCPWM_MCLV2_PIM_DualShunt_R2015b_InternalOpAmp/Compute Voltage applied Within Alpha Beta Space1 ==
  Gain : Inport
  CosSin : Inport  Port=2
  DC Bus Voltage : Inport  Port=3
  Abs : Abs
  Delay : Delay  DelayLength=1  InitialCondition=0
  Product1 : Product  RndMeth=Zero  OutDataTypeStr=Inherit: Same as first input
  Product3 : Product  OutMin=[-24]  OutMax=[24]  RndMeth=Zero  OutDataTypeStr=Inherit: Same as first input
  ValphaBeta : Outport
  wires:
  Abs/1 -> Product1/2
  Gain/1 -> Abs/1
  CosSin/1 -> Delay/1
  Product3/1 -> ValphaBeta/1
  Product1/1 -> Product3/1
  DC Bus Voltage/1 -> Product3/2
  Delay/1 -> Product1/1

== system PIC32MK_MCPWM_MCLV2_PIM_DualShunt_R2015b_InternalOpAmp/Invert Current Sign For reversed rotation1 ==
  Gain : Inport
  "Iab " : Inport  Port=2
  Compare To Zero1 : simulink/Logic and Bit Operations/Compare To Zero  relop=>=  OutDataTypeStr=boolean
  Gain4 : Gain  Gain=-1  RndMeth=Zero  SaturateOnIntegerOverflow=on  OutDataTypeStr=Inherit: Same as input
  Switch3 : Switch  Criteria=u2 ~= 0  Threshold=250
  "Iab_ " : Outport
  wires:
  "Iab "/1 -> Gain4/1, Switch3/1
  Gain/1 -> Compare To Zero1/1
  Switch3/1 -> "Iab_ "/1
  Compare To Zero1/1 -> Switch3/2
  Gain4/1 -> Switch3/3

== system PIC32MK_MCPWM_MCLV2_PIM_DualShunt_R2015b_InternalOpAmp/MCLV-V2 PIC32MK Pinout ==
  note: MCLV-V2 Board - PIC32MK PIM
      |
      | MCLV Board | PIN
      | ========================
      | PGC | RB6 | PGC2
      | PGD | RB5 | PGD2
  note: MCLV-V2 Board - PIC32MK PIM
      |
      | MCLV Board | PIN
      | ========================
      | UART_Rx | RA8
      | UART_Tx | RC8
  note: MCLV-V2 Board - PIC32MK PIM
      |
      | MCLV Board | PIN
      | ========================
      | HALLA | RC9
      | HALLB | RE14
      | HALLC | RA14
      | HOME | RG6
  note: MCLV-V2 Board - PIC32MK PIM
      |
      | MCLV Board | PIN
      | ========================
      | Vref | AN34 | RF10
      | Pot | AN15 | RE15
      | VBUS | AN10 | RA12
      | REC_NEUTR | AN18 | RG7
      |
      | Ia | AN24| RA4 Phase Current-1
      | Ib | AN9 | RA11 Phase Current-2
      | IBUS | AN25| RB7 Bus Current
  note: MCLV-V2 Board - PIC32MK PIM
      |
      | MCLV Board | PIN
      | ========================
      | PWM1H | RB14
      | PWM1L | RB15
      |
      | PWM2H | RB12
      | PWM2L | RB13
      |
      | PWM3H | RB10
      | PWM3L | RB11
      |
      | MC_FAULT | RB4 - FLT15
  note: MCLV-V2 Board - PIC32MK PIM
      |
      | MCLV Board | PIN
      | ========================
      | LED1 | RF5
      | LED2 | RG15
      | ---------------------------|-------------------
      | SW1 | RG1
      | SW2 | RC7
  note: PINOUT - MCLV-V2 Board - PIC32MK PIM

== system PIC32MK_MCPWM_MCLV2_PIM_DualShunt_R2015b_InternalOpAmp/OPEN Loop Startup sequence ==
  Constant1 : Constant  Value=149*2^-32  OutDataTypeStr=fixdt(0,32,32)  SampleTime=.00005
  Delay : Delay  DelayLength=1  InitialCondition=0
  Delay2 : Delay  DelayLength=1  InitialCondition=0
  Saturation : Saturate  UpperLimit=149*2^-32*3/.00005  LowerLimit=0
  Sum : Sum  Inputs=|++  AccumDataTypeStr=fixdt(0,32,32)  OutDataTypeStr=Inherit: Same as accumulator  RndMeth=Simplest
  Sum1 : Sum  Inputs=|++  AccumDataTypeStr=fixdt(0,32,32)  OutDataTypeStr=Inherit: Same as accumulator  RndMeth=Simplest
  Out1 : Outport
  wires:
  Delay/1 -> Sum/2
  Sum/1 -> Saturation/1  "Startup Ramp"
  Constant1/1 -> Sum/1
  Sum1/1 -> Out1/1, Delay2/1  "qAngle"
  Delay2/1 -> Sum1/2
  Saturation/1 -> Delay/1, Sum1/1

== system PIC32MK_MCPWM_MCLV2_PIM_DualShunt_R2015b_InternalOpAmp/Scale ==
  In1 : Inport
  Data Type Conversion : DataTypeConversion  OutDataTypeStr=fixdt(1,32,31)
  Data Type Conversion1 : DataTypeConversion  OutDataTypeStr=fixdt(0,32,32)  ConvertRealWorld=Stored Integer (SI)
  Rate Transition2 : RateTransition
  Phase shift : Outport
  wires:
  In1/1 -> Data Type Conversion/1
  Data Type Conversion/1 -> Data Type Conversion1/1
  Data Type Conversion1/1 -> Rate Transition2/1
  Rate Transition2/1 -> Phase shift/1
